simulink model "simu"  (R2015a)
settings: Solver=ode45  StartTime=0.0  StopTime=3  FixedStep=0.01  RelTol=1e-3
values from neighbouring files (symbols this model uses):
  theta0 = [0 0 0 0 0]'    [main.m]
settings Model: Creator=andreas  LastModifiedBy=andreas

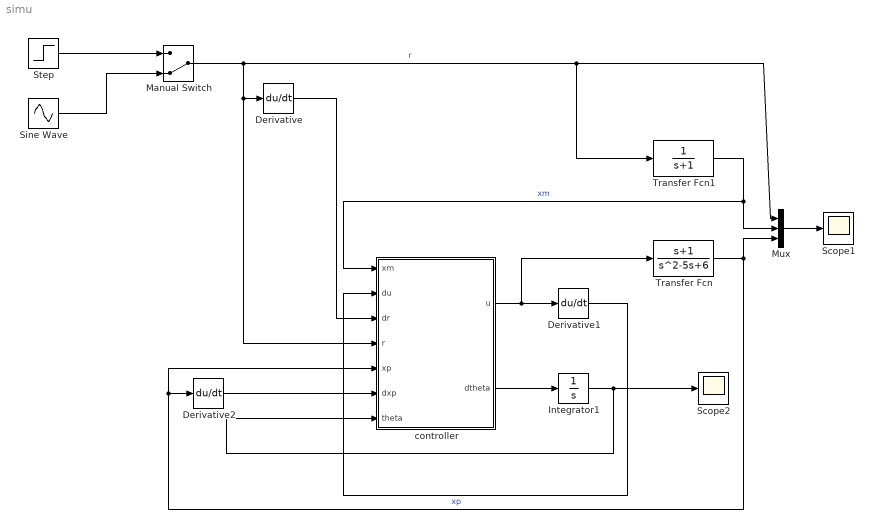
== system simu ==
  Derivative : Derivative
  Derivative1 : Derivative
  Derivative2 : Derivative
  Integrator1 : Integrator  InitialCondition=theta0
  Manual Switch : ManualSwitch  CurrentSetting=0
  Mux : Mux  Inputs=3
  Scope1 : Scope
      settings: ShowLegends=on  YMin=0  YMax=1.4
  Scope2 : Scope
      settings: ShowLegends=on  YMin=-4.5e+07  YMax=2.5e+07  SaveName=ScopeData2
  Sine Wave : Sin  SampleTime=0
  Step : Step  SampleTime=0
  Transfer Fcn : TransferFcn  Numerator=[1 1]  Denominator=[1 -5 6]
  Transfer Fcn1 : TransferFcn  Denominator=[1 1]
  controller : MATLAB Function  TreatAsAtomicUnit=on
  wires:
  controller/2(dtheta) -> Integrator1/1
  Mux/1 -> Scope1/1
  Step/1 -> Manual Switch/1
  Sine Wave/1 -> Manual Switch/2
  Integrator1/1 -> Scope2/1, controller/7(theta)
  Manual Switch/1 -> Derivative/1, controller/4(r), Transfer Fcn1/1, Mux/1  "r"
  Derivative/1 -> controller/3(dr)
  controller/1(u) -> Transfer Fcn/1, Derivative1/1
  Transfer Fcn1/1 -> Mux/2, controller/1(xm)  "xm"
  Derivative1/1 -> controller/2(du)
  Transfer Fcn/1 -> Mux/3, controller/5(xp), Derivative2/1  "xp"
  Derivative2/1 -> controller/6(dxp)

== matlab function simu/controller ==
  data: xm input; du input; u output; dr input; r input; xp input; dxp input; theta input; dtheta output; gamma parameter
function [u, dtheta] = controller(xm, du, dr, r, xp, dxp, theta, gamma)
%#codegen

e = xp - xm;

phi = [dr, r, dxp, xp, du]';

u = theta'*phi;

dtheta = -gamma*phi*e;
